simulink model "Mass_Spring_Damper_System2"  (R2025b)
settings: Solver=FixedStepAuto  StartTime=0.0  StopTime=tspan  FixedStep=dt  RelTol=1e-3
values from neighbouring files (symbols this model uses):
  b = transpose(1:10)    [TestLoop.m]    (also in init.m = rand()*(dampingRange(2)-dampingRange(1))+dampingRange(1))
  dt_data = round((dt_data_target/dt))*dt    [init.m]
  k = transpose(1:10)    [TestLoop.m]    (also in init.m = rand()*(stiffnessRange(2)-stiffnessRange(1))+stiffnessRange()
  m = transpose(1:10)    [TestLoop.m]    (also in init.m = rand()*(massRange(2)-massRange(1))+massRange(1))
  v0 = transpose(1:10)    [TestLoop.m]    (also in init.m = rand()*(velocityRange(2)-velocityRange(1))+velocityRange(1))
  x0 = transpose(1:10)    [TestLoop.m]    (also in init.m = rand()*(positionRange(2)-positionRange(1))+positionRange(1))
settings Model: Creator=ajosh  LastModifiedBy=bochaocai

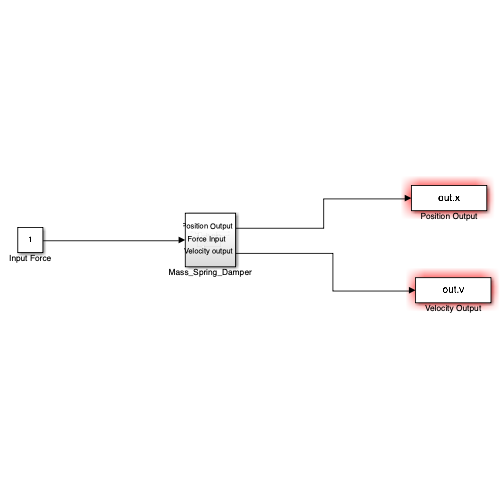
[thumbnail: Simulink's stored preview of the top-level diagram]
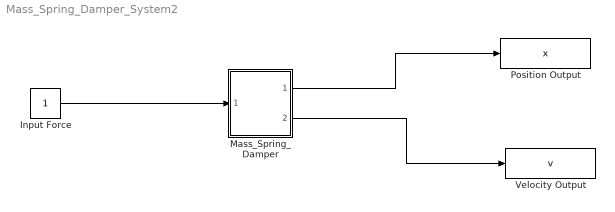
== system Mass_Spring_Damper_System2 ==
  Input Force : Constant
  Mass_Spring_Damper : Subsystem
  Position Output : ToWorkspace  VariableName=x  SaveFormat=Timeseries  SampleTime=dt_data
  Velocity Output : ToWorkspace  VariableName=v  SaveFormat=Timeseries  SampleTime=dt_data
  wires:
  Input Force/1 -> Mass_Spring_Damper/1(Force Input)
  Mass_Spring_Damper/1(Position Output) -> Position Output/1
  Mass_Spring_Damper/2(Velocity output) -> Velocity Output/1

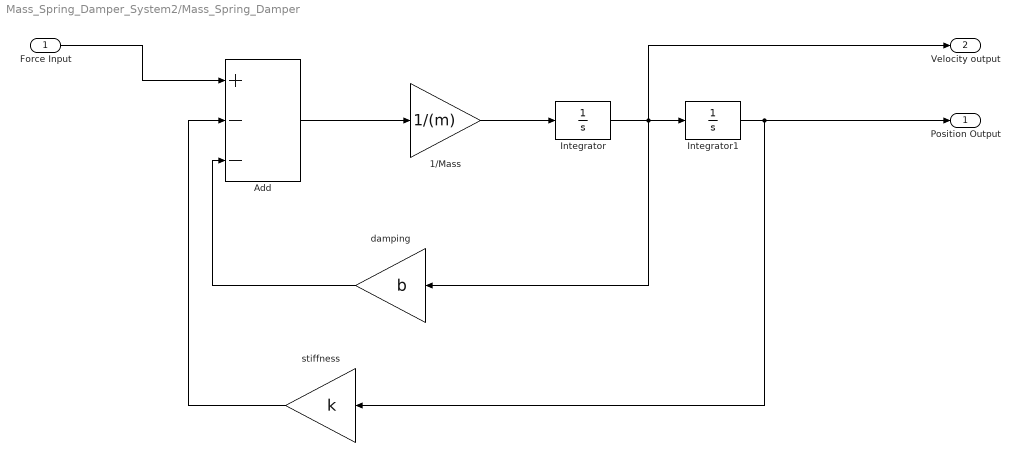
== system Mass_Spring_Damper_System2/Mass_Spring_Damper ==
  Force Input : Inport
  1/Mass : Gain  Gain=1/(m)
  Add : Sum  Inputs=+--
  Integrator : Integrator  InitialCondition=v0
  Integrator1 : Integrator  InitialCondition=x0
  damping : Gain  Gain=b
  stiffness : Gain  Gain=k
  Position Output : Outport
  Velocity output : Outport  Port=2
  wires:
  Integrator/1 -> Velocity output/1, damping/1, Integrator1/1
  1/Mass/1 -> Integrator/1
  Integrator1/1 -> Position Output/1, stiffness/1
  damping/1 -> Add/3
  stiffness/1 -> Add/2
  Add/1 -> 1/Mass/1
  Force Input/1 -> Add/1
